simulink model "maglev_test"  (R2018b)
settings: Solver=ode1  StartTime=0.0  StopTime=70  FixedStep=0.0005  RelTol=1e-3
libraries: simulink x1
settings Model: Creator=zhou-  LastModifiedBy=zhou-

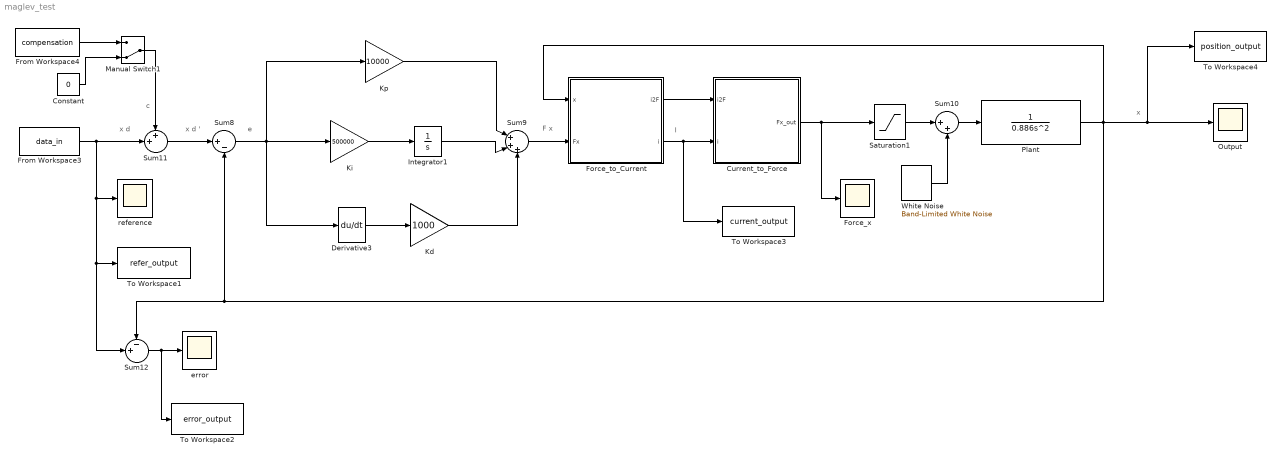
== system maglev_test ==
  note: x d
  note: x d '
  note: c
  note: e
  note: F x
  note: I
  note: x
  Constant : Constant  Value=0
  Current_to_Force : MATLAB Function  TreatAsAtomicUnit=on
  Derivative3 : Derivative
  Force_to_Current : MATLAB Function  TreatAsAtomicUnit=on
  Force_x : Scope
  From Workspace3 : FromWorkspace  VariableName=data_in  SampleTime=0
  From Workspace4 : FromWorkspace  VariableName=compensation  SampleTime=0
  Integrator1 : Integrator
  Kd : Gain  Gain=1000
  Ki : Gain  Gain=500000
  Kp : Gain  Gain=10000
  Manual Switch1 : ManualSwitch  CurrentSetting=0
  Output : Scope
  Plant : TransferFcn  Denominator=[0.886 0 0]
  Saturation1 : Saturate  UpperLimit=10  LowerLimit=-10
  Sum10 : Sum  Inputs=|++
  Sum11 : Sum  Inputs=++|
  Sum12 : Sum  Inputs=-+|
  Sum8 : Sum  Inputs=|+-
  Sum9 : Sum  Inputs=|+++
  To Workspace1 : ToWorkspace  VariableName=refer_output  SaveFormat=Timeseries  SampleTime=-1
  To Workspace2 : ToWorkspace  VariableName=error_output  SaveFormat=Timeseries  SampleTime=-1
  To Workspace3 : ToWorkspace  VariableName=current_output  SaveFormat=Timeseries  SampleTime=-1
  To Workspace4 : ToWorkspace  VariableName=position_output  SaveFormat=Timeseries  SampleTime=-1
  White Noise : simulink/Sources/Band-Limited White Noise  Cov=[0.000000]  Ts=0.0005  seed=[23341]
  error : Scope
  reference : Scope
  wires:
  Sum8/1 -> Derivative3/1, Kp/1, Ki/1
  Ki/1 -> Integrator1/1
  Derivative3/1 -> Kd/1
  Kd/1 -> Sum9/3
  Integrator1/1 -> Sum9/2
  Kp/1 -> Sum9/1
  Saturation1/1 -> Sum10/1
  Current_to_Force/1(Fx_out) -> Saturation1/1, Force_x/1
  White Noise/1 -> Sum10/2
  Sum10/1 -> Plant/1
  Sum9/1 -> Force_to_Current/2(Fx)
  Force_to_Current/1(i2F) -> Current_to_Force/1(i2F)
  Force_to_Current/2(i) -> To Workspace3/1, Current_to_Force/2(i)
  From Workspace4/1 -> Manual Switch1/1
  Constant/1 -> Manual Switch1/2
  Sum11/1 -> Sum8/1
  Plant/1 -> Sum8/2, Sum12/1, Force_to_Current/1(x), To Workspace4/1, Output/1
  From Workspace3/1 -> Sum12/2, To Workspace1/1, reference/1, Sum11/2
  Manual Switch1/1 -> Sum11/1
  Sum12/1 -> To Workspace2/1, error/1

== matlab function maglev_test/Force_to_Current ==
  data: i2F output; x input; Fx input; i output
function [i2F,i] = fcn_f_to_i(x,Fx)

i = zeros(25,1);
i2F = zeros(6,25);

%%% 基本参数
B0=0.45;%B0常数
S=2.5*10^-6;%导线截面积
hc=0.0165;%线圈高度
r_in=0.005;%线圈内径
r_out=0.03;%线圈外径
t=0.0375;%磁钢阵列极距

%%% 为了减少重复计算引入的常数
K0=4*B0/sqrt(2)/S;
k=sqrt(2)*pi/t;

% 推力系数矩阵，在磁浮平面电机设计阶段就可率先计算出来
U=[0 -2.7387 0 0;
   0 0 0 -2.7387;
   2.7387 0 2.7387 0;
   0 0 0 2.4986e-04;
   0 -2.4986e-04 0 0;
   0 0 0 0];

% 所有线圈在基坐标系中的位置
b_C = cell(5,5);
for i = 1:5
    for j = 1:5
        b_C{i,j}= [(2*j-1)*r_out;(2*i-1)*r_out;0];
    end
end

% 磁钢阵列在基坐标系中的位置
b_My = 0.14;% 只考虑x方向上的运动，y方向运动看做一个固定值，随机取一个有意义的值
b_Mz = 0.001;% 气隙高度，取1mm
b_M = [x;b_My;b_Mz];

% 计算其电流→推力的映射矩阵(//只让完全位于磁钢阵列下方的线圈工作，减少边缘效应）
Rot_z_45 = [sqrt(2)/2 sqrt(2)/2 0;-sqrt(2)/2 sqrt(2)/2 0;0 0 1]; %从MCS到RMCS的旋转矩阵
R_theta = [Rot_z_45' zeros(3);zeros(3) Rot_z_45']; % 6*6的旋转矩阵

% 电流→力的映射矩阵,初始化为空矩阵，每个线圈增加一个6*1的列向量到该矩阵中
i2F_mapping_matrix = zeros(6,25);

% 对每个线圈分别进行计算
for i = 1:5
    for j = 1:5
%         if b_C{i,j}(1)>(b_M(1)+4*t-r_out) || b_C{i,j}(1)<(b_M(1)-4*t+r_out) || b_C{i,j}(2)>(b_M(2)+4*t-r_out) || b_C{i,j}(2)<(b_M(2)-4*t+r_out)
%             i2F_mapping_matrix(:,5*(i-1)+j) = zeros(6,1);
%         
%         else
            rm_C = Rot_z_45*(b_C{i,j}-b_M);% 计算线圈在RMCS中的位置
            
            % 计算位置矢量
            e = [cos(k*rm_C(1));sin(k*rm_C(1));cos(k*rm_C(2));cos(k*rm_C(2))];
        
            % 计算移轴转换矩阵
            Y = [ 1 0 0 0 0 0;
                  0 1 0 0 0 0;
                  0 0 1 0 0 0;
                  0 -rm_C(3) rm_C(2) 1 0 0;
                  rm_C(3) 0 -rm_C(1) 0 1 0;
                  -rm_C(2) rm_C(1) 0 0 0 1;];
        
            % 更新电流→力的映射矩阵
            i2F_mapping_matrix(:,5*(i-1)+j) = exp(k*rm_C(3)).*R_theta*Y*U*e;
%         end
    end
end

% 计算最终的电流分配结果
desired_wrench = [Fx;0;44.1;0;0;0];
cal_i = pinv(i2F_mapping_matrix)*desired_wrench;

% 输出结果
i = cal_i;
i2F = i2F_mapping_matrix;

== matlab function maglev_test/Current_to_Force ==
  data: i2F input; i input; Fx_out output
function Fx_out = fcn_i_to_f(i2F,i)
Fx_out = i2F(1,:)*i;
